simulink model "MoHinhCoastDownChung"  (R2024b)
settings: Solver=VariableStepAuto  StartTime=0.0  RelTol=1e-3  AbsTol=1e-3  EnableMultiTasking=on
values from neighbouring files (symbols this model uses):
  a = 0.2657    [CodeSosanhCoastdownCumdongluc.m]    (also in CodeSosanhCoastdownCumtaotai.m = 0.0601)
  b = 6.7129    [CodeSosanhCoastdownCumdongluc.m]    (also in CodeSosanhCoastdownCumtaotai.m = 8.2494)
  initial = data(1,4)*2*pi()/60    [CodeSosanhCoastdownCumdongluc.m]    (also in CodeSosanhCoastdownCumtaotai.m = data(1,2)*2*pi()/60)
  J = 0.2412    [CodeSosanhCoastdownCumdongluc.m]    (also in CodeSosanhCoastdownCumtaotai.m = 1.2576)
  Tst = 15    [CodeSosanhCoastdownCumdongluc.m]    (also in CodeSosanhCoastdownCumtaotai.m = 2)
undefined symbols (not defined in the file or in its folder): rad, s
libraries: aerolibconvert2 x1
settings Model: Creator=Admin  LastModifiedBy=Legion
settings SolverCC: AutoScaleAbsTol=off  AlgebraicLoopSolver=TrustRegion  MaxZcPerStep=1
settings DataIOCC: LimitDataPoints=on  MaxDataPoints=10000
settings OptimizationCC: ReuseModelBlockBuffer=off  LifeSpan=inf
settings DebuggingCC: UnconnectedInputMsg=warning  UnconnectedOutputMsg=warning  UnconnectedLineMsg=warning  AllowSymbolicDim=off  SubsystemReferenceDiagnosticForUnitTest=warning  SFUnexpectedBacktrackingDiag=warning  SFNoUnconditionalDefaultTransitionDiag=warning  SFExecutionAtInitializationDiag=none  ArithmeticOperatorsInVariantConditions=warning
settings ModelReferenceCC: EnableRefExpFcnMdlSchedulingChecks=on
settings SFSimCC: SimUseLocalCustomCode=off  CustomCodeUndefinedFunction=UseInterfaceOnly
settings RTWCC: RTWUseLocalCustomCode=off  GPUComputeCapability=3.5  DLArmComputeVersion=19.05
settings CodeAppCC: StateflowObjectComments=on
settings GRTTargetCC: TargetLangStandard=C89/C90 (ANSI)
settings ConfigComp: CovMetricSettings=dw  CovSaveCumulativeToWorkspaceVar=on  CovSaveSingleToWorkspaceVar=on  CovExternalEMLEnable=off  CovSFcnEnable=off
settings SimscapeCC: SimscapeLogType=all  SimscapeLogSimulationStatistics=on  SimscapeLogDataHistory=10000

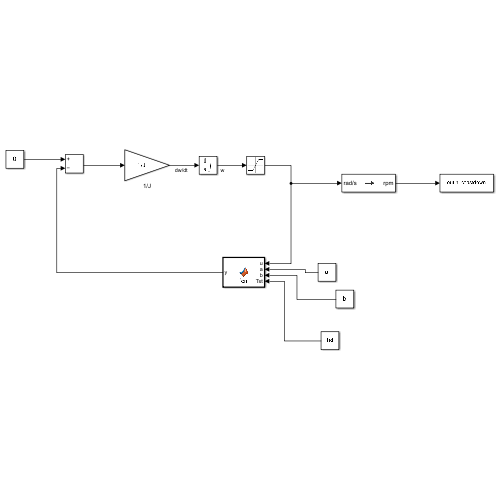
[thumbnail: Simulink's stored preview of the top-level diagram]
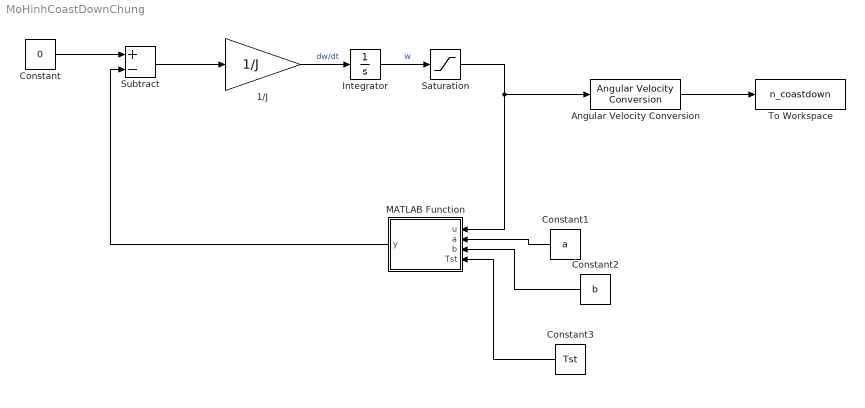
== system MoHinhCoastDownChung ==
  1/J : Gain  Gain=1/J
  Angular Velocity Conversion : aerolibconvert2/Angular Velocity Conversion  IU=rad/s  OU=rpm
  Constant : Constant  Value=0
  Constant1 : Constant  Value=a
  Constant2 : Constant  Value=b
  Constant3 : Constant  Value=Tst
  Integrator : Integrator  InitialCondition=initial  LimitOutput=on  LowerSaturationLimit=0
  MATLAB Function : MATLAB Function  TreatAsAtomicUnit=on
  Saturation : Saturate  UpperLimit=inf  LowerLimit=0
  Subtract : Sum  Inputs=+-
  To Workspace : ToWorkspace  VariableName=n_coastdown  SaveFormat=Timeseries  SampleTime=-1
  wires:
  Constant/1 -> Subtract/1
  Subtract/1 -> 1/J/1
  1/J/1 -> Integrator/1  "dw/dt"
  MATLAB Function/1(y) -> Subtract/2
  Constant1/1 -> MATLAB Function/2(a)
  Constant2/1 -> MATLAB Function/3(b)
  Integrator/1 -> Saturation/1  "w"
  Saturation/1 -> Angular Velocity Conversion/1, MATLAB Function/1(u)
  Constant3/1 -> MATLAB Function/4(Tst)
  Angular Velocity Conversion/1 -> To Workspace/1

== matlab function MoHinhCoastDownChung/MATLAB Function ==
  data: u input; y output; a input; b input; Tst input
function y = fcn(u,a,b,Tst)
y=0.0362*(a*u+b)*Tst;
